simulink model "sim_vereinfacht"  (R2021b)
settings: Solver=VariableStepAuto  StartTime=0.0  StopTime=10.0  RelTol=1e-3
undefined symbols (not defined in the file or in its folder): Rohr2, waermekapazitaet_luft, waermekapazitaet_wasser_gasfoermig
libraries: Feuchtesimulation_Lib x5
settings Model: Creator=q552088  LastModifiedBy=q552088

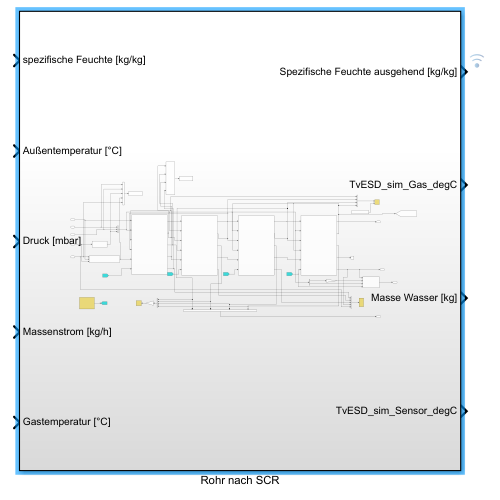
[thumbnail: Simulink's stored preview of the top-level diagram]
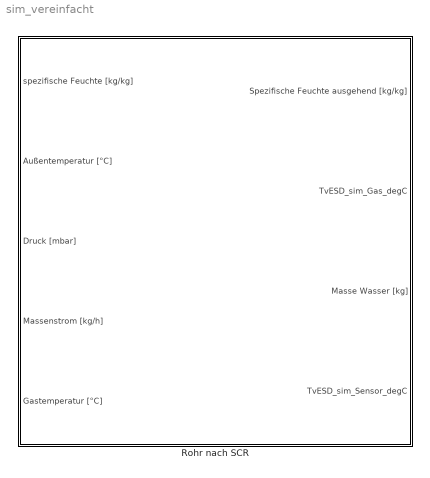
== system sim_vereinfacht ==
  Rohr nach SCR : Subsystem

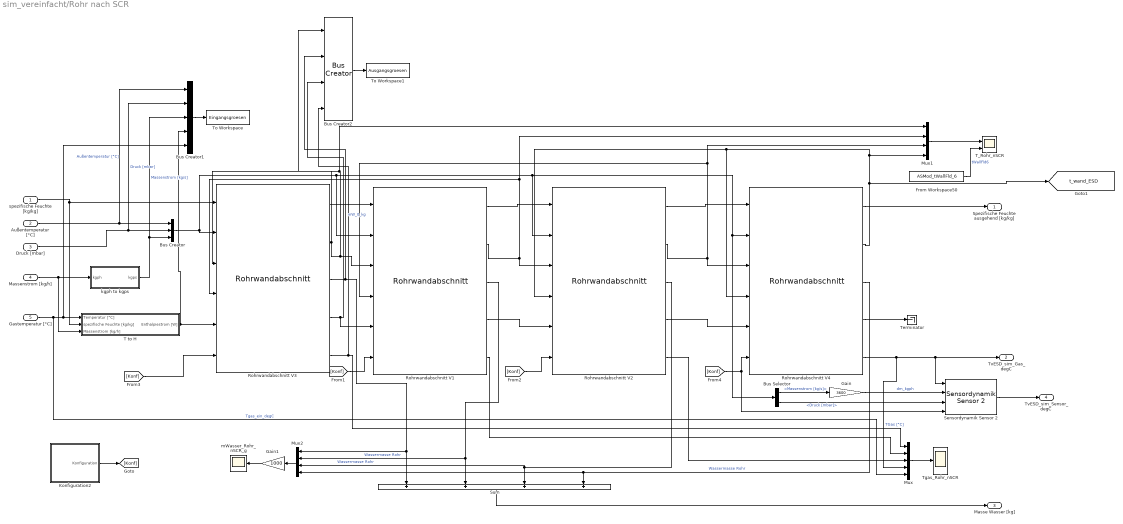
== system sim_vereinfacht/Rohr nach SCR ==
  spezifische Feuchte [kg/kg] : Inport
  Außentemperatur [°C] : Inport  Port=2
  Druck [mbar] : Inport  Port=3
  Massenstrom [kg/h] : Inport  Port=4
  Gastemperatur [°C] : Inport  Port=5
  Bus Creator : BusCreator  Inputs=3
  Bus Creator1 : BusCreator  Inputs=5
  Bus Creator2 : BusCreator  Inputs=4
  Bus Selector : BusSelector  OutputSignals=Massenstrom [kg/s],Druck [mbar]
  From Workspace50 : FromWorkspace  VariableName=ASMod_tWallFld_6  OutputAfterFinalValue=Holding final value
  Gain : Gain  Gain=3600
  Gain1 : Gain  Gain=1000
  Konfiguration2 : Subsystem
  Mux : Mux  Inputs=5
  Mux1 : Mux
  Mux2 : Mux
  Rohrwandabschnitt V{1..4} (4 alike) : Feuchtesimulation_Lib/Rohrwandabschnitt  SystemSampleTime=-1  VariantActivationTime=update diagram  Latency=0  AutoFrameSizeCalculation=off
  Sensordynamik Sensor 2 : Feuchtesimulation_Lib/Sensordynamik Sensor 2  SystemSampleTime=-1  VariantActivationTime=update diagram  Latency=0  AutoFrameSizeCalculation=off
  Sum : Sum  Inputs=++++
  T to H : Subsystem
  T_Rohr_nSCR : Scope  NumInputPorts=2
  Terminator : Terminator
  Tgas_Rohr_nSCR : Scope
  To Workspace : ToWorkspace  VariableName=Eingangsgroesen  SaveFormat=Structure With Time  SampleTime=-1
  To Workspace1 : ToWorkspace  VariableName=Ausgangsgroesen  SaveFormat=Structure With Time  SampleTime=-1
  kgph to kgps : Subsystem
  mWasser_Rohr_nSCR_g : Scope
  Spezifische Feuchte ausgehend [kg/kg] : Outport  VectorParamsAs1DForOutWhenUnconnected=off
  TvESD_sim_Gas_degC : Outport  Port=2  VectorParamsAs1DForOutWhenUnconnected=off
  Masse Wasser [kg] : Outport  Port=3  VectorParamsAs1DForOutWhenUnconnected=off
  TvESD_sim_Sensor_degC : Outport  Port=4  VectorParamsAs1DForOutWhenUnconnected=off
  tag scope: t_wand_ESD=global
  wires:
  spezifische Feuchte [kg/kg]/1 -> Rohrwandabschnitt V3/1, T to H/2(spezifische Feuchte [kg/kg])
  Massenstrom [kg/h]/1 -> T to H/3(Massenstrom [kg/h]), kgph to kgps/1(kgph)
  Konfiguration2/1(Konfiguration) -> [Konf]
  Gastemperatur [°C]/1 -> T to H/1(Temperatur [°C]), Bus Creator1/5, Mux/5  "Tgas_ein_degC"
  Rohrwandabschnitt V3/1 -> Rohrwandabschnitt V1/1
  Rohrwandabschnitt V1/1 -> Rohrwandabschnitt V2/1
  Rohrwandabschnitt V2/1 -> Rohrwandabschnitt V4/1
  Rohrwandabschnitt V3/4 -> Bus Creator2/3, Rohrwandabschnitt V1/5
  Rohrwandabschnitt V1/4 -> Rohrwandabschnitt V2/5
  Rohrwandabschnitt V2/4 -> Rohrwandabschnitt V4/5
  [Konf] -> Rohrwandabschnitt V1/6
  [Konf] -> Rohrwandabschnitt V2/6
  [Konf] -> Rohrwandabschnitt V3/6
  Außentemperatur [°C]/1 -> Bus Creator1/1, Bus Creator/1  "Außentemperatur [°C]"
  kgph to kgps/1(kgps) -> Bus Creator/3, Bus Creator1/3  "Massenstrom [kg/s]"
  Druck [mbar]/1 -> Bus Creator/2, Bus Creator1/2  "Druck [mbar]"
  T to H/1(Enthalpiestrom [W]) -> Bus Creator1/4, Rohrwandabschnitt V3/5
  Rohrwandabschnitt V3/2 -> Bus Creator2/1, Mux1/1, Rohrwandabschnitt V3/3, Rohrwandabschnitt V1/3
  Rohrwandabschnitt V1/2 -> Mux1/2, Rohrwandabschnitt V3/4, Rohrwandabschnitt V2/3
  Rohrwandabschnitt V2/2 -> Mux1/3, Rohrwandabschnitt V1/4, Rohrwandabschnitt V4/3
  Rohrwandabschnitt V4/2 -> [t_wand_ESD], Mux1/4, Rohrwandabschnitt V4/4, Rohrwandabschnitt V2/4
  Rohrwandabschnitt V4/1 -> Spezifische Feuchte ausgehend [kg/kg]/1
  Rohrwandabschnitt V3/3 -> Bus Creator2/2, Sum/1, Mux2/1  "mW_0_kg"
  Rohrwandabschnitt V1/3 -> Mux2/2, Sum/2  "Wassermasse Rohr"
  Rohrwandabschnitt V2/3 -> Sum/3, Mux2/3  "Wassermasse Rohr"
  Rohrwandabschnitt V4/3 -> Mux2/4, Sum/4  "Wassermasse Rohr"
  Sum/1 -> Masse Wasser [kg]/1
  Rohrwandabschnitt V2/5 -> Mux/3
  Rohrwandabschnitt V3/5 -> Bus Creator2/4, Mux/1
  Rohrwandabschnitt V1/5 -> Mux/2
  Mux/1 -> Tgas_Rohr_nSCR/1
  Rohrwandabschnitt V4/5 -> Mux/4, Sensordynamik Sensor 2/1, TvESD_sim_Gas_degC/1  "TGas [°C]"
  Mux1/1 -> T_Rohr_nSCR/1
  Rohrwandabschnitt V4/4 -> Terminator/1
  From Workspace50/1 -> T_Rohr_nSCR/2  "tWallFld6"
  [Konf] -> Sensordynamik Sensor 2/4, Rohrwandabschnitt V4/6
  Bus Selector/2 -> Sensordynamik Sensor 2/3  "<Druck [mbar]>"
  Bus Selector/1 -> Gain/1  "<Massenstrom [kg/s]>"
  Gain/1 -> Sensordynamik Sensor 2/2  "dm_kgph"
  Sensordynamik Sensor 2/1 -> TvESD_sim_Sensor_degC/1
  Bus Creator/1 -> Rohrwandabschnitt V1/2, Rohrwandabschnitt V2/2, Bus Selector/1, Rohrwandabschnitt V4/2, Rohrwandabschnitt V3/2
  Gain1/1 -> mWasser_Rohr_nSCR_g/1
  Mux2/1 -> Gain1/1
  Bus Creator1/1 -> To Workspace/1
  Bus Creator2/1 -> To Workspace1/1

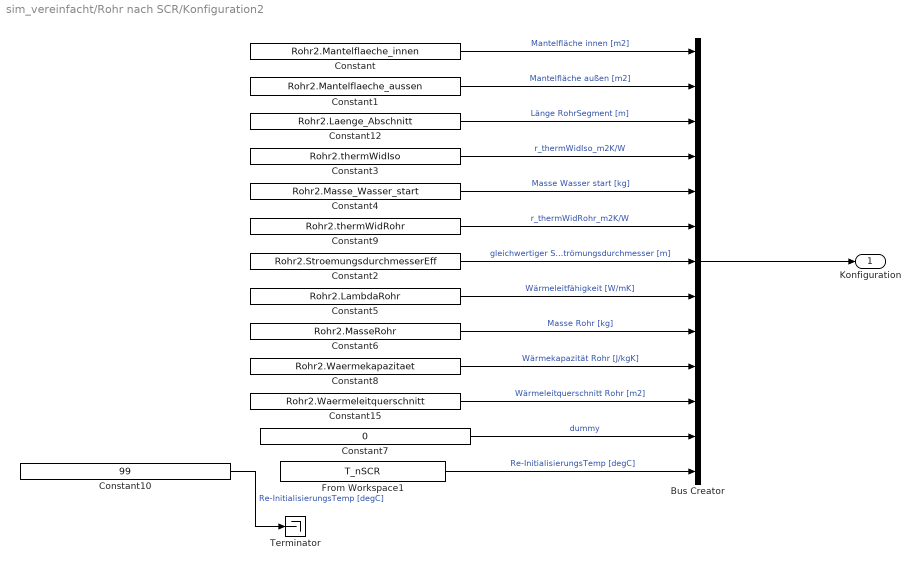
== system sim_vereinfacht/Rohr nach SCR/Konfiguration2 ==
  Bus Creator : BusCreator  Inputs=13
  Constant : Constant  Value=Rohr2.Mantelflaeche_innen
  Constant1 : Constant  Value=Rohr2.Mantelflaeche_aussen
  Constant10 : Constant  Value=99
  Constant12 : Constant  Value=Rohr2.Laenge_Abschnitt
  Constant15 : Constant  Value=Rohr2.Waermeleitquerschnitt
  Constant2 : Constant  Value=Rohr2.StroemungsdurchmesserEff
  Constant3 : Constant  Value=Rohr2.thermWidIso
  Constant4 : Constant  Value=Rohr2.Masse_Wasser_start
  Constant5 : Constant  Value=Rohr2.LambdaRohr
  Constant6 : Constant  Value=Rohr2.MasseRohr
  Constant7 : Constant  Value=0
  Constant8 : Constant  Value=Rohr2.Waermekapazitaet
  Constant9 : Constant  Value=Rohr2.thermWidRohr
  From Workspace1 : FromWorkspace  VariableName=T_nSCR
  Terminator : Terminator
  Konfiguration : Outport  VectorParamsAs1DForOutWhenUnconnected=off
  wires:
  Bus Creator/1 -> Konfiguration/1
  Constant/1 -> Bus Creator/1  "Mantelfläche innen [m2]"
  Constant1/1 -> Bus Creator/2  "Mantelfläche außen [m2]"
  Constant4/1 -> Bus Creator/5  "Masse Wasser start [kg]"
  Constant12/1 -> Bus Creator/3  "Länge RohrSegment [m]"
  Constant15/1 -> Bus Creator/11  "Wärmeleitquerschnitt Rohr [m2]"
  Constant2/1 -> Bus Creator/7  "gleichwertiger Strömungsdurchmesser [m]"
  Constant5/1 -> Bus Creator/8  "Wärmeleitfähigkeit [W/mK]"
  Constant6/1 -> Bus Creator/9  "Masse Rohr [kg]"
  Constant8/1 -> Bus Creator/10  "Wärmekapazität Rohr [J/kgK]"
  From Workspace1/1 -> Bus Creator/13  "Re-InitialisierungsTemp [degC]"
  Constant3/1 -> Bus Creator/4  "r_thermWidIso_m2K/W"
  Constant9/1 -> Bus Creator/6  "r_thermWidRohr_m2K/W"
  Constant7/1 -> Bus Creator/12  "dummy"
  Constant10/1 -> Terminator/1  "Re-InitialisierungsTemp [degC]"

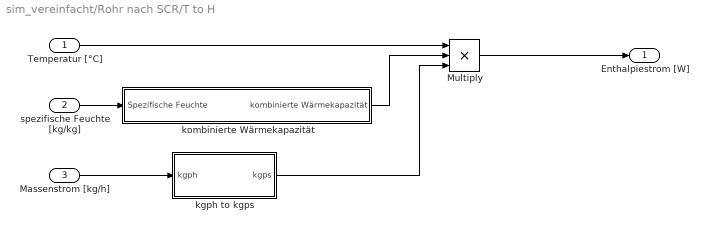
== system sim_vereinfacht/Rohr nach SCR/T to H ==
  Temperatur [°C] : Inport
  spezifische Feuchte [kg/kg] : Inport  Port=2
  Massenstrom [kg/h] : Inport  Port=3
  Multiply : Product  Inputs=3
  kgph to kgps : Subsystem
  kombinierte Wärmekapazität : Subsystem
  Enthalpiestrom [W] : Outport  VectorParamsAs1DForOutWhenUnconnected=off
  wires:
  Massenstrom [kg/h]/1 -> kgph to kgps/1(kgph)
  Temperatur [°C]/1 -> Multiply/1
  spezifische Feuchte [kg/kg]/1 -> kombinierte Wärmekapazität/1(Spezifische Feuchte)
  Multiply/1 -> Enthalpiestrom [W]/1
  kombinierte Wärmekapazität/1(kombinierte Wärmekapazität) -> Multiply/2
  kgph to kgps/1(kgps) -> Multiply/3

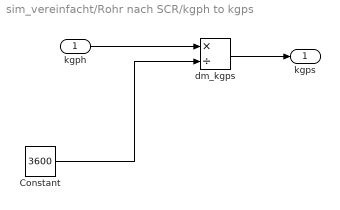
== system sim_vereinfacht/Rohr nach SCR/kgph to kgps ==
  kgph : Inport
  Constant : Constant  Value=3600
  dm_kgps : Product  Inputs=*/
  kgps : Outport  VectorParamsAs1DForOutWhenUnconnected=off
  wires:
  dm_kgps/1 -> kgps/1
  kgph/1 -> dm_kgps/1
  Constant/1 -> dm_kgps/2

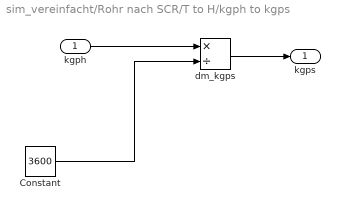
== system sim_vereinfacht/Rohr nach SCR/T to H/kgph to kgps ==
  kgph : Inport
  Constant : Constant  Value=3600
  dm_kgps : Product  Inputs=*/
  kgps : Outport  VectorParamsAs1DForOutWhenUnconnected=off
  wires:
  dm_kgps/1 -> kgps/1
  kgph/1 -> dm_kgps/1
  Constant/1 -> dm_kgps/2

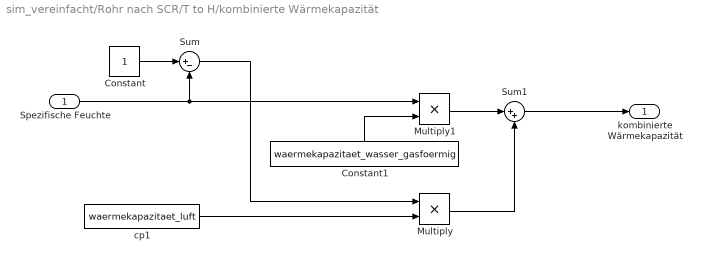
== system sim_vereinfacht/Rohr nach SCR/T to H/kombinierte Wärmekapazität ==
  Spezifische Feuchte : Inport
  Constant : Constant
  Constant1 : Constant  Value=waermekapazitaet_wasser_gasfoermig
  Multiply : Product
  Multiply1 : Product
  Sum : Sum  Inputs=|+-
  Sum1 : Sum  Inputs=|++
  cp1 : Constant  Value=waermekapazitaet_luft
  kombinierte Wärmekapazität : Outport  VectorParamsAs1DForOutWhenUnconnected=off
  wires:
  Multiply/1 -> Sum1/2
  Sum/1 -> Multiply/1
  Constant/1 -> Sum/1
  Spezifische Feuchte/1 -> Sum/2, Multiply1/1
  Constant1/1 -> Multiply1/2
  cp1/1 -> Multiply/2
  Multiply1/1 -> Sum1/1
  Sum1/1 -> kombinierte Wärmekapazität/1
